simulink library "KP"  (R2016a)
settings: Solver=ode45  StartTime=0.0  StopTime=10.0  RelTol=1e-3
libraries: simulink x1
settings Model: Creator=KDFX Team  LastModifiedBy=KDFX Team
settings DataIOCC: LimitDataPoints=on
settings DebuggingCC: AllowSymbolicDim=off

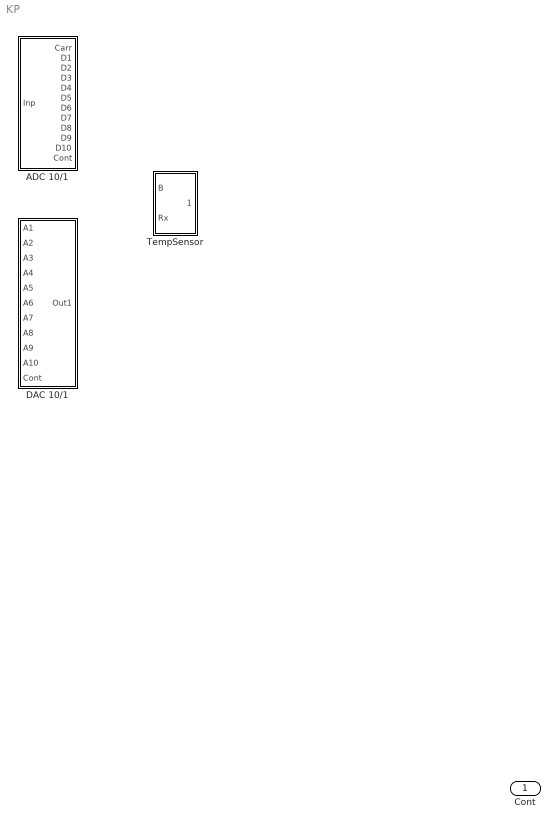
== system KP ==
  Cont : Inport
  ADC 10/1 : Subsystem
  DAC 10/1 : Subsystem
  TempSensor : Subsystem

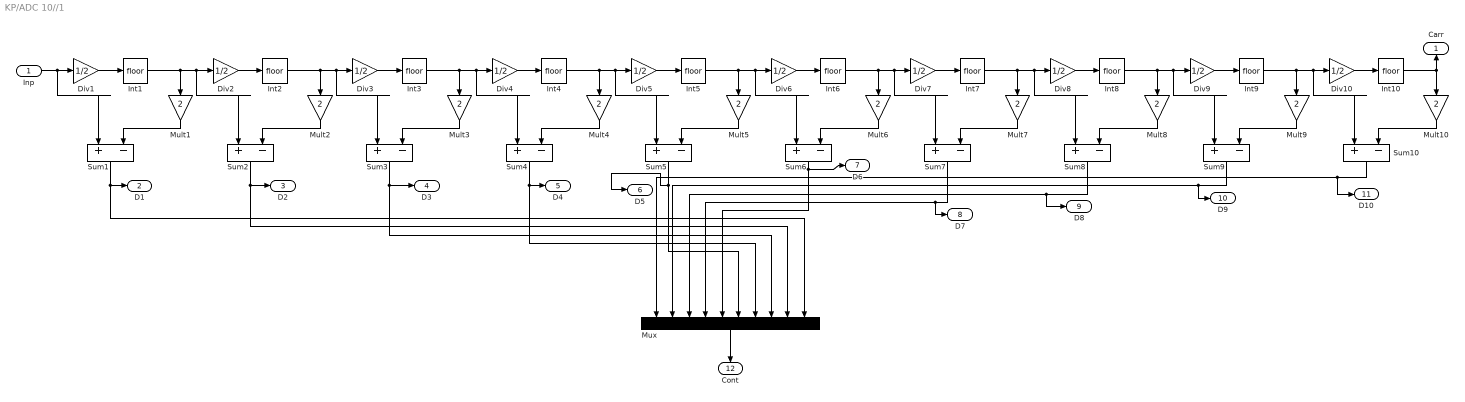
== system KP/ADC 10//1 ==
  Inp : Inport
  Div{1..10} (10 alike) : Gain  Gain=1/2  SaturateOnIntegerOverflow=on  OutDataTypeStr=Inherit: Same as input  ParamDataTypeStr=Inherit: Same as input
  Int{1..10} (10 alike) : Rounding
  Mult{1..10} (10 alike) : Gain  Gain=2  SaturateOnIntegerOverflow=on  OutDataTypeStr=Inherit: Same as input  ParamDataTypeStr=Inherit: Same as input
  Mux : Mux  Inputs=10
  Sum{1..10} (10 alike) : Sum  Inputs=|+-  SaturateOnIntegerOverflow=on
  Carr : Outport  InitialOutput=0
  D1 : Outport  Port=2  InitialOutput=0
  D2 : Outport  Port=3  InitialOutput=0
  D3 : Outport  Port=4  InitialOutput=0
  D4 : Outport  Port=5  InitialOutput=0
  D5 : Outport  Port=6  InitialOutput=0
  D6 : Outport  Port=7  InitialOutput=0
  D7 : Outport  Port=8  InitialOutput=0
  D8 : Outport  Port=9  InitialOutput=0
  D9 : Outport  Port=10  InitialOutput=0
  D10 : Outport  Port=11  InitialOutput=0
  Cont : Outport  Port=12  InitialOutput=0
  wires:
  Sum1/1 -> Mux/10, D1/1
  Sum2/1 -> Mux/9, D2/1
  Sum3/1 -> Mux/8, D3/1
  Sum4/1 -> Mux/7, D4/1
  Sum5/1 -> Mux/6, D5/1
  Sum6/1 -> Mux/5, D6/1
  Sum7/1 -> Mux/4, D7/1
  Sum8/1 -> Mux/3, D8/1
  Sum9/1 -> Mux/2, D9/1
  Sum10/1 -> Mux/1, D10/1
  Mux/1 -> Cont/1
  Int9/1 -> Mult9/1, Div10/1, Sum10/1
  Mult10/1 -> Sum10/2
  Int10/1 -> Mult10/1, Carr/1
  Div10/1 -> Int10/1
  Mult9/1 -> Sum9/2
  Div9/1 -> Int9/1
  Int7/1 -> Mult7/1, Div8/1, Sum8/1
  Mult8/1 -> Sum8/2
  Int8/1 -> Mult8/1, Div9/1, Sum9/1
  Div8/1 -> Int8/1
  Mult7/1 -> Sum7/2
  Div7/1 -> Int7/1
  Int5/1 -> Mult5/1, Div6/1, Sum6/1
  Mult6/1 -> Sum6/2
  Int6/1 -> Mult6/1, Sum7/1, Div7/1
  Div6/1 -> Int6/1
  Mult5/1 -> Sum5/2
  Div5/1 -> Int5/1
  Int3/1 -> Mult3/1, Div4/1, Sum4/1
  Mult4/1 -> Sum4/2
  Int4/1 -> Mult4/1, Div5/1, Sum5/1
  Div4/1 -> Int4/1
  Mult3/1 -> Sum3/2
  Div3/1 -> Int3/1
  Int1/1 -> Mult1/1, Div2/1, Sum2/1
  Mult2/1 -> Sum2/2
  Int2/1 -> Mult2/1, Sum3/1, Div3/1
  Div2/1 -> Int2/1
  Mult1/1 -> Sum1/2
  Inp/1 -> Div1/1, Sum1/1
  Div1/1 -> Int1/1

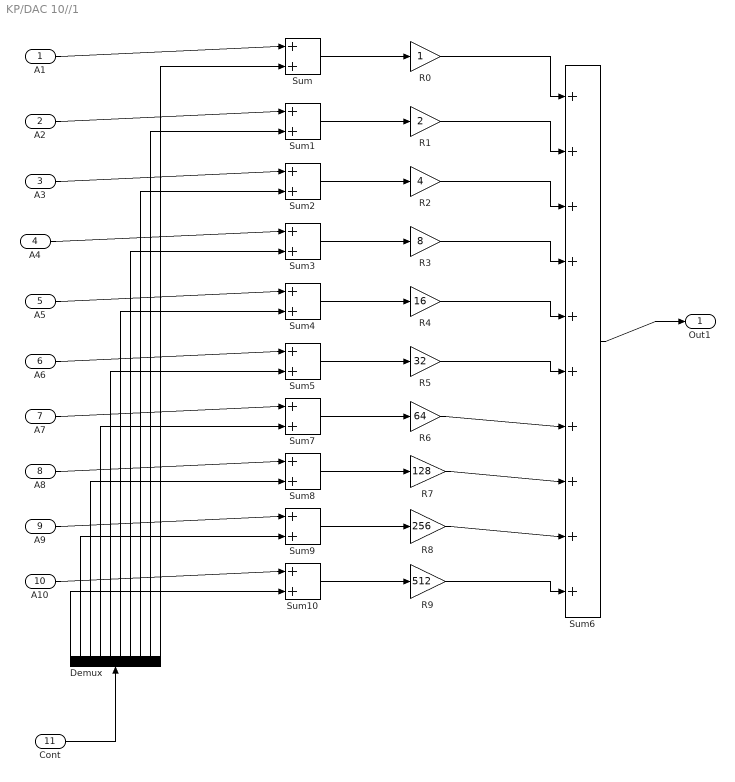
== system KP/DAC 10//1 ==
  A1 : Inport
  A2 : Inport  Port=2
  A3 : Inport  Port=3
  A4 : Inport  Port=4
  A5 : Inport  Port=5
  A6 : Inport  Port=6
  A7 : Inport  Port=7
  A8 : Inport  Port=8
  A9 : Inport  Port=9
  A10 : Inport  Port=10
  Cont : Inport  Port=11
  Demux : Demux  Outputs=10
  R0 : Gain  SaturateOnIntegerOverflow=on  OutDataTypeStr=Inherit: Same as input  ParamDataTypeStr=Inherit: Same as input
  R1 : Gain  Gain=2  SaturateOnIntegerOverflow=on  OutDataTypeStr=Inherit: Same as input  ParamDataTypeStr=Inherit: Same as input
  R2 : Gain  Gain=4  SaturateOnIntegerOverflow=on  OutDataTypeStr=Inherit: Same as input  ParamDataTypeStr=Inherit: Same as input
  R3 : Gain  Gain=8  SaturateOnIntegerOverflow=on  OutDataTypeStr=Inherit: Same as input  ParamDataTypeStr=Inherit: Same as input
  R4 : Gain  Gain=16  SaturateOnIntegerOverflow=on  OutDataTypeStr=Inherit: Same as input  ParamDataTypeStr=Inherit: Same as input
  R5 : Gain  Gain=32  SaturateOnIntegerOverflow=on  OutDataTypeStr=Inherit: Same as input  ParamDataTypeStr=Inherit: Same as input
  R6 : Gain  Gain=64  SaturateOnIntegerOverflow=on  OutDataTypeStr=Inherit: Same as input  ParamDataTypeStr=Inherit: Same as input
  R7 : Gain  Gain=128  SaturateOnIntegerOverflow=on  OutDataTypeStr=Inherit: Same as input  ParamDataTypeStr=Inherit: Same as input
  R8 : Gain  Gain=256  SaturateOnIntegerOverflow=on  OutDataTypeStr=Inherit: Same as input  ParamDataTypeStr=Inherit: Same as input
  R9 : Gain  Gain=512  SaturateOnIntegerOverflow=on  OutDataTypeStr=Inherit: Same as input  ParamDataTypeStr=Inherit: Same as input
  Sum{,1..5,7..10} (10 alike) : Sum  Inputs=|++  SaturateOnIntegerOverflow=on  InputSameDT=on  OutDataTypeStr=Inherit: Same as first input
  Sum6 : Sum  Inputs=|++++++++++  SaturateOnIntegerOverflow=on  InputSameDT=on  OutDataTypeStr=Inherit: Same as first input
  Out1 : Outport  InitialOutput=0
  wires:
  R5/1 -> Sum6/6
  Sum2/1 -> R2/1
  Sum4/1 -> R4/1
  R3/1 -> Sum6/4
  R2/1 -> Sum6/3
  R1/1 -> Sum6/2
  Sum5/1 -> R5/1
  Sum3/1 -> R3/1
  Sum/1 -> R0/1
  Sum6/1 -> Out1/1
  R4/1 -> Sum6/5
  Sum1/1 -> R1/1
  A6/1 -> Sum5/1
  A3/1 -> Sum2/1
  A4/1 -> Sum3/1
  A5/1 -> Sum4/1
  A2/1 -> Sum1/1
  A1/1 -> Sum/1
  Sum7/1 -> R6/1
  R6/1 -> Sum6/7
  A7/1 -> Sum7/1
  Sum8/1 -> R7/1
  R7/1 -> Sum6/8
  A8/1 -> Sum8/1
  Sum9/1 -> R8/1
  R8/1 -> Sum6/9
  A9/1 -> Sum9/1
  Sum10/1 -> R9/1
  R9/1 -> Sum6/10
  A10/1 -> Sum10/1
  R0/1 -> Sum6/1
  Cont/1 -> Demux/1
  Demux/1 -> Sum10/2
  Demux/2 -> Sum9/2
  Demux/3 -> Sum8/2
  Demux/4 -> Sum7/2
  Demux/5 -> Sum5/2
  Demux/6 -> Sum4/2
  Demux/7 -> Sum3/2
  Demux/8 -> Sum2/2
  Demux/9 -> Sum1/2
  Demux/10 -> Sum/2

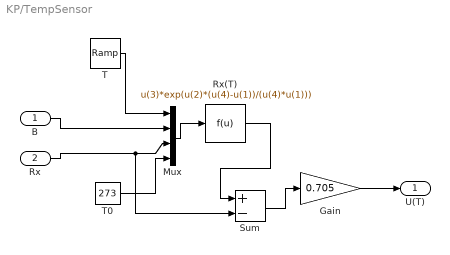
== system KP/TempSensor ==
  B : Inport
  Rx : Inport  Port=2
  Gain : Gain  Gain=0.705  SaturateOnIntegerOverflow=on  OutDataTypeStr=Inherit: Same as input  ParamDataTypeStr=Inherit: Same as input
  Mux : Mux
  Rx(T) : Fcn  Expr=u(3)*exp(u(2)*(u(4)-u(1))/(u(4)*u(1)))
  Sum : Sum  Inputs=+-  SaturateOnIntegerOverflow=on  InputSameDT=on  OutDataTypeStr=Inherit: Same as first input
  T : simulink/Sources/Ramp  slope=0.16  start=0  X0=288
  T0 : Constant  Value=273  SampleTime=0
  U(T) : Outport  InitialOutput=0
  wires:
  Rx(T)/1 -> Sum/1
  Gain/1 -> U(T)/1
  Sum/1 -> Gain/1
  Rx/1 -> Sum/2, Mux/3
  T0/1 -> Mux/4
  T/1 -> Mux/1
  B/1 -> Mux/2
  Mux/1 -> Rx(T)/1
